simulink model "simu_maquina_papel"  (R2018a)
settings: Solver=VariableStepAuto  StartTime=0.0  StopTime=20  RelTol=1e-9
values from neighbouring files (symbols this model uses):
  Kr = Kr_0/K(1)    [control_maquina_papel.m]
  T = 1    [control_maquina_papel.m]
libraries: cstblocks x1
settings Model: Creator=pablo  LastModifiedBy=pablo

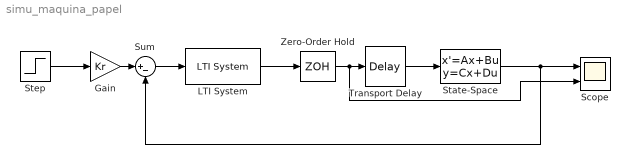
== system simu_maquina_papel ==
  Gain : Gain  Gain=Kr
  LTI System : cstblocks/LTI System  sys=Control  IC=[]
  Scope : Scope  NumInputPorts=2
  State-Space : StateSpace  A=-1  D=0  InitialCondition=0
  Step : Step  SampleTime=0
  Sum : Sum  Inputs=|+-
  Transport Delay : TransportDelay  DelayTime=2.5
  Zero-Order Hold : ZeroOrderHold  SampleTime=T
  wires:
  Transport Delay/1 -> State-Space/1
  LTI System/1 -> Zero-Order Hold/1
  Sum/1 -> LTI System/1
  Gain/1 -> Sum/1
  Zero-Order Hold/1 -> Scope/2, Transport Delay/1
  State-Space/1 -> Sum/2, Scope/1
  Step/1 -> Gain/1
